simulink model "PID_with_PreFilter"  (R2018b)
settings: Solver=FixedStepAuto  StartTime=0.0  StopTime=5  FixedStep=0.001  RelTol=1e-3
settings Model: Creator=hp0016  LastModifiedBy=hp0016

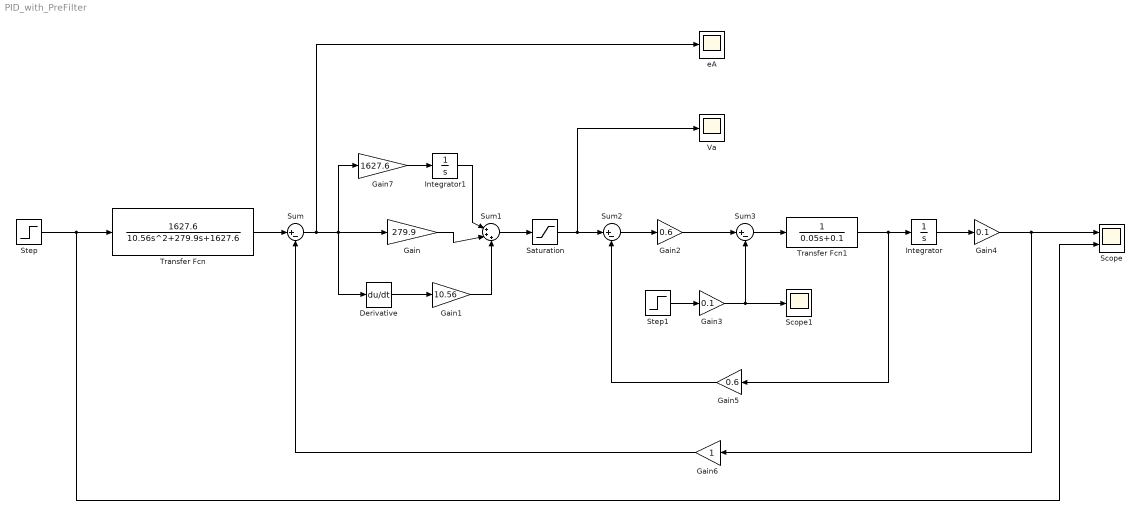
== system PID_with_PreFilter ==
  Derivative : Derivative
  Gain : Gain  Gain=279.9
  Gain1 : Gain  Gain=10.56
  Gain2 : Gain  Gain=0.6
  Gain3 : Gain  Gain=0.1
  Gain4 : Gain  Gain=0.1
  Gain5 : Gain  Gain=0.6
  Gain6 : Gain
  Gain7 : Gain  Gain=1627.6
  Integrator : Integrator
  Integrator1 : Integrator
  Saturation : Saturate  UpperLimit=125  LowerLimit=-125
  Scope : Scope  NumInputPorts=2
  Scope1 : Scope
  Step : Step  SampleTime=0
  Step1 : Step  Time=3  After=180  SampleTime=0
  Sum : Sum  Inputs=|+-
  Sum1 : Sum  Inputs=|+++
  Sum2 : Sum  Inputs=|+-
  Sum3 : Sum  Inputs=|+-
  Transfer Fcn : TransferFcn  Numerator=[1627.6]  Denominator=[10.56 279.9 1627.6]
  Transfer Fcn1 : TransferFcn  Denominator=[0.05 0.1]
  Va : Scope
  eA : Scope
  wires:
  Gain3/1 -> Sum3/2, Scope1/1
  Step1/1 -> Gain3/1
  Step/1 -> Transfer Fcn/1, Scope/2
  Transfer Fcn/1 -> Sum/1
  Sum/1 -> Gain7/1, Gain/1, Derivative/1, eA/1
  Derivative/1 -> Gain1/1
  Sum1/1 -> Saturation/1
  Saturation/1 -> Va/1, Sum2/1
  Gain5/1 -> Sum2/2
  Sum2/1 -> Gain2/1
  Gain2/1 -> Sum3/1
  Sum3/1 -> Transfer Fcn1/1
  Transfer Fcn1/1 -> Gain5/1, Integrator/1
  Integrator/1 -> Gain4/1
  Gain4/1 -> Gain6/1, Scope/1
  Gain6/1 -> Sum/2
  Gain7/1 -> Integrator1/1
  Integrator1/1 -> Sum1/1
  Gain/1 -> Sum1/2
  Gain1/1 -> Sum1/3
